simulink model "IFM_ModelComposer"  (R2024b)
settings: Solver=VariableStepAuto  StartTime=0.0  StopTime=2e-4  RelTol=1e-3
PreLoadFcn:
  | addpath('../Matlab_Scripts/','-end')
  | addpath('../System_Inputs/','-end')
  | System
undefined symbols (not defined in the file): Fs, time_delays, xlfda_numerator
libraries: hdlBasic x77, hdlDSPIP x4, hdlUtilities x1, vmcUtilities x1
settings Model: Creator=fsy  LastModifiedBy=fsydere

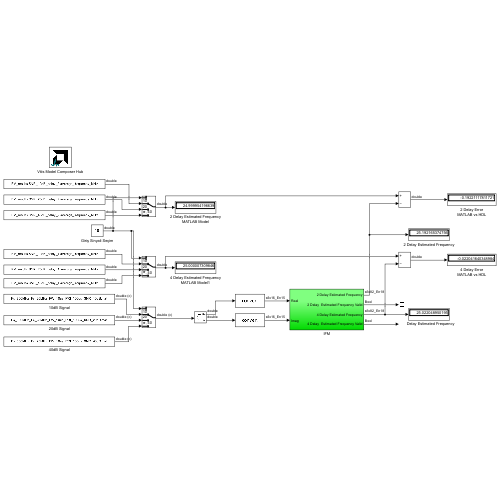
[thumbnail: Simulink's stored preview of the top-level diagram]
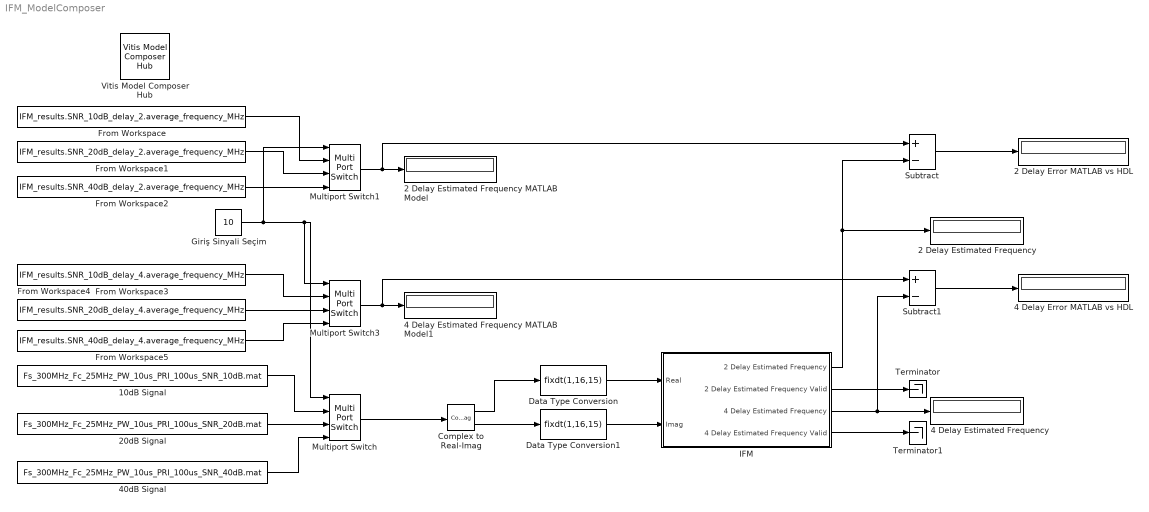
== system IFM_ModelComposer ==
  10dB Signal : FromFile  FileName=Fs_300MHz_Fc_25MHz_PW_10us_PRI_100us_SNR_10dB.mat  SampleTime=1/Fs
  2 Delay Error MATLAB vs HDL : Display
  2 Delay Estimated Frequency : Display
  2 Delay Estimated Frequency MATLAB Model : Display
  20dB Signal : FromFile  FileName=Fs_300MHz_Fc_25MHz_PW_10us_PRI_100us_SNR_20dB.mat  SampleTime=1/Fs
  4 Delay Error MATLAB vs HDL : Display
  4 Delay Estimated Frequency : Display
  4 Delay Estimated Frequency MATLAB Model1 : Display
  40dB Signal : FromFile  FileName=Fs_300MHz_Fc_25MHz_PW_10us_PRI_100us_SNR_40dB.mat  SampleTime=1/Fs
  Complex to Real-Imag : ComplexToRealImag
  Data Type Conversion : DataTypeConversion  OutDataTypeStr=fixdt(1,16,15)  RndMeth=Round
  Data Type Conversion1 : DataTypeConversion  OutDataTypeStr=fixdt(1,16,15)  RndMeth=Round
  From Workspace : FromWorkspace  VariableName=IFM_results.SNR_10dB_delay_2.average_frequency_MHz  SampleTime=1/Fs
  From Workspace1 : FromWorkspace  VariableName=IFM_results.SNR_20dB_delay_2.average_frequency_MHz  SampleTime=1/Fs
  From Workspace2 : FromWorkspace  VariableName=IFM_results.SNR_40dB_delay_2.average_frequency_MHz  SampleTime=1/Fs
  From Workspace3 : FromWorkspace  VariableName=IFM_results.SNR_10dB_delay_4.average_frequency_MHz  SampleTime=1/Fs
  From Workspace4 : FromWorkspace  VariableName=IFM_results.SNR_20dB_delay_4.average_frequency_MHz  SampleTime=1/Fs
  From Workspace5 : FromWorkspace  VariableName=IFM_results.SNR_40dB_delay_4.average_frequency_MHz  SampleTime=1/Fs
  Giriş Sinyali Seçim : Constant  Value=10  SampleTime=1/Fs
  IFM : Subsystem
  Multiport Switch : MultiPortSwitch  DataPortOrder=Specify indices  DataPortIndices={10,20,40}  OutDataTypeStr=double  SaturateOnIntegerOverflow=off  InputSameDT=off
  Multiport Switch1 : MultiPortSwitch  DataPortOrder=Specify indices  DataPortIndices={10,20,40}  OutDataTypeStr=double  SaturateOnIntegerOverflow=off  InputSameDT=off
  Multiport Switch3 : MultiPortSwitch  DataPortOrder=Specify indices  DataPortIndices={10,20,40}  OutDataTypeStr=double  SaturateOnIntegerOverflow=off  InputSameDT=off
  Subtract : Sum  Inputs=+-
  Subtract1 : Sum  Inputs=+-
  Terminator : Terminator
  Terminator1 : Terminator
  Vitis Model Composer Hub : vmcUtilities/Vitis Model Composer Hub  Tag=genX  CodeGeneration=off  SubsystemName=IFM  BlockHierPath=IFM_ModelComposer/IFM  CompilationType=HDLCompilation  SubsystemType=HDLNode  ExportTypeV2=IP Catalog  StartColumn=1  NumberOfColumns=1  TargetDirectory=./netlist  exportDesign=off  analyzeDesign=on  validateDesignOnHw=off  ExportType=AI Engines  IpVendor=xilinx.com  IpLibrary=hls  IpVersion=1.0  IpHWLanguage=Verilog  AieCompilerOptions={}  AieSimulatorOptions={}  CreateTestbench=on  TestbenchStackSize=10  RunRtlSim=off  RunCSim=off  RunAieSim=off  AieSimTimeout=50000  RunAieSimProfiling=off  LaunchVitisAnalyzer=off  PlotOutput=off  RunX86Sim=off  X86SimTimeout=10  GenHwImage=off  GenLibadfXo=off  GenHwValidationCode=off  PlatformType=Not Specified  HwSystemType=Baremetal  HwValidationTarget=hw  ProjDevice=Zynq UltraScale+ ZCU102 Evaluation Board (xczu9eg-ffvb1156-2-e)  ProjDevicePart=xczu9eg-ffvb1156-2-e  AIEType=None  SamplePeriod=-1  ClockFrequency=200  DataPathParallelism=1  xilinxfamily=zynquplus  part=xczu9eg  speed=-2-e  package=ffvb1156  directory=./netlist\ip\IFM\src  testbench=on  incr_netlist=off  synthesis_tool=Vivado  clock_wrapper=Clock Enables  dbl_ovrd=According to Block Masks  dcm_input_clock_period=10  sysclk_period=1e9/Fs  simulink_period=1/Fs  eval_field=0  IPInfoJsonString="{\"DUTSubsystemName\":\"IFM\",\"HDLSubsystem\":{\"SubsystemName\":\"IFM\",\"IPName\":\"IFM\",\"IPLibrary\":\"VMC\",\"IPVendor\":\"FSY\",\"IPVersion\":\"1.0\",\"TargetDirectory\":\"./netlist\",\"SubsystemDir\":\"./netlist\\\\ip\\\\IFM\",\"FreqHz\":\"300000000\"},\"SubsystemTag\":\"HDLNode\"}"  LogFileName=C:\Users\fsydere\Workspace\IFM\Model_Composer\netlist\model_composer.log  NThreads=10  IPConfigFile=C:\Users\fsydere\AppData\Local\Temp\vmctmp-16672868257368253290\IFM_ModelComposer_ipconfig.json
  wires:
  From Workspace/1 -> Multiport Switch1/2
  10dB Signal/1 -> Multiport Switch/2
  From Workspace5/1 -> Multiport Switch3/4
  From Workspace1/1 -> Multiport Switch1/3
  From Workspace2/1 -> Multiport Switch1/4
  Giriş Sinyali Seçim/1 -> Multiport Switch/1, Multiport Switch3/1, Multiport Switch1/1
  From Workspace3/1 -> Multiport Switch3/2
  From Workspace4/1 -> Multiport Switch3/3
  20dB Signal/1 -> Multiport Switch/3
  40dB Signal/1 -> Multiport Switch/4
  Multiport Switch1/1 -> Subtract/1, 2 Delay Estimated Frequency MATLAB Model/1
  Multiport Switch3/1 -> Subtract1/1, 4 Delay Estimated Frequency MATLAB Model1/1
  Multiport Switch/1 -> Complex to Real-Imag/1
  Complex to Real-Imag/1 -> Data Type Conversion/1
  Complex to Real-Imag/2 -> Data Type Conversion1/1
  Data Type Conversion/1 -> IFM/1(Real)
  Data Type Conversion1/1 -> IFM/2(Imag)
  Subtract1/1 -> 4 Delay Error MATLAB vs HDL/1
  IFM/1(2 Delay Estimated Frequency) -> 2 Delay Estimated Frequency/1, Subtract/2
  IFM/2(2 Delay Estimated Frequency Valid) -> Terminator/1
  IFM/3(4 Delay Estimated Frequency) -> Subtract1/2, 4 Delay Estimated Frequency/1
  IFM/4(4 Delay Estimated Frequency Valid) -> Terminator1/1
  Subtract/1 -> 2 Delay Error MATLAB vs HDL/1

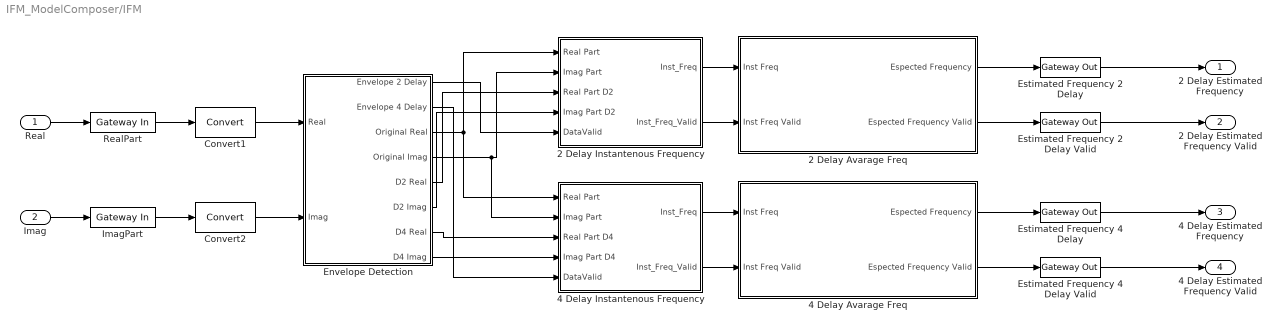
== system IFM_ModelComposer/IFM ==
  Real : Inport
  Imag : Inport  Port=2
  2 Delay Avarage Freq : Subsystem
  2 Delay Instantenous Frequency : Subsystem
  4 Delay Avarage Freq : Subsystem
  4 Delay Instantenous Frequency : Subsystem
  Convert1 : hdlBasic/Convert  gui_display_data_type=Fixed-point  arith_type=Signed (2's comp)  n_bits=16  bin_pt=15  float_type=Single  exp_bits=8  fraction_bits=24  quantization=Truncate  overflow=Wrap  en=off  latency=0  pipeline=off  XmcBlockStatus=1  maskContainerNames=group2  block_type=convert  block_config=sysgen:Convert_config  block_width=595  block_height=885
  Convert2 : hdlBasic/Convert  gui_display_data_type=Fixed-point  arith_type=Signed (2's comp)  n_bits=16  bin_pt=15  float_type=Single  exp_bits=8  fraction_bits=24  quantization=Truncate  overflow=Wrap  en=off  latency=0  pipeline=off  XmcBlockStatus=1  maskContainerNames=group2  block_type=convert  block_config=sysgen:Convert_config  block_width=595  block_height=885
  Envelope Detection : Subsystem
  Estimated Frequency 2 Delay : hdlBasic/Gateway Out  inherit_from_input=on  bool_to_boolean=off  hdl_port=on  rows=1  columns=1  UseAsDAC=off  DACChannel='1'  interface=None  automatic_assignment=on  address_offset=hex2dec('00')  intf_name=''  intf_description=''  timing_constraint=None  locs_specified=off  LOCs={}  io_standard={}  XmcBlockStatus=1  maskContainerNames=group4  block_type=gatewayout  block_config=sysgen:gateway_out_config  block_width_w=590  block_height_w=620  block_width=620  block_height=750
  Estimated Frequency 2 Delay Valid : hdlBasic/Gateway Out  inherit_from_input=on  bool_to_boolean=off  hdl_port=on  rows=1  columns=1  UseAsDAC=off  DACChannel='1'  interface=None  automatic_assignment=on  address_offset=hex2dec('00')  intf_name=''  intf_description=''  timing_constraint=None  locs_specified=off  LOCs={}  io_standard={}  XmcBlockStatus=1  maskContainerNames=group4  block_type=gatewayout  block_config=sysgen:gateway_out_config  block_width_w=590  block_height_w=620  block_width=620  block_height=750
  Estimated Frequency 4 Delay : hdlBasic/Gateway Out  inherit_from_input=on  bool_to_boolean=off  hdl_port=on  rows=1  columns=1  UseAsDAC=off  DACChannel='1'  interface=None  automatic_assignment=on  address_offset=hex2dec('00')  intf_name=''  intf_description=''  timing_constraint=None  locs_specified=off  LOCs={}  io_standard={}  XmcBlockStatus=1  maskContainerNames=group4  block_type=gatewayout  block_config=sysgen:gateway_out_config  block_width_w=590  block_height_w=620  block_width=620  block_height=750
  Estimated Frequency 4 Delay Valid : hdlBasic/Gateway Out  inherit_from_input=on  bool_to_boolean=off  hdl_port=on  rows=1  columns=1  UseAsDAC=off  DACChannel='1'  interface=None  automatic_assignment=on  address_offset=hex2dec('00')  intf_name=''  intf_description=''  timing_constraint=None  locs_specified=off  LOCs={}  io_standard={}  XmcBlockStatus=1  maskContainerNames=group4  block_type=gatewayout  block_config=sysgen:gateway_out_config  block_width_w=590  block_height_w=620  block_width=620  block_height=750
  ImagPart : hdlBasic/Gateway In  gui_display_data_type=Fixed-point  arith_type=Signed (2's comp)  n_bits=16  bin_pt=15  preci_type=Single  exp_width=8  frac_width=24  rows=1  columns=1  quantization=Truncate  overflow=Wrap  period=1/Fs  UseAsADC=off  ADCChannel='1'  interface=None  automatic_assignment=on  address_offset=hex2dec('00')  intf_name=''  intf_description=''  default_value=0  timing_constraint=None  locs_specified=off  LOCs={}  io_standard={}  inherit_from_input=off  hdl_port=on  XmcBlockStatus=1  maskContainerNames=group4  block_type=gatewayin  block_config=sysgen:gateway_in_config  block_width_w=590  block_height_w=620  block_width=640  block_height=850
  RealPart : hdlBasic/Gateway In  gui_display_data_type=Fixed-point  arith_type=Signed (2's comp)  n_bits=16  bin_pt=15  preci_type=Single  exp_width=8  frac_width=24  rows=1  columns=1  quantization=Truncate  overflow=Wrap  period=1/Fs  UseAsADC=off  ADCChannel='1'  interface=None  automatic_assignment=on  address_offset=hex2dec('00')  intf_name=''  intf_description=''  default_value=0  timing_constraint=None  locs_specified=off  LOCs={}  io_standard={}  inherit_from_input=off  hdl_port=on  XmcBlockStatus=1  maskContainerNames=group4  block_type=gatewayin  block_config=sysgen:gateway_in_config  block_width_w=590  block_height_w=620  block_width=640  block_height=850
  2 Delay Estimated Frequency : Outport
  2 Delay Estimated Frequency Valid : Outport  Port=2
  4 Delay Estimated Frequency : Outport  Port=3
  4 Delay Estimated Frequency Valid : Outport  Port=4
  wires:
  2 Delay Avarage Freq/1(Espected Frequency) -> Estimated Frequency 2 Delay/1
  Real/1 -> RealPart/1
  ImagPart/1 -> Convert2/1
  Imag/1 -> ImagPart/1
  RealPart/1 -> Convert1/1
  Convert2/1 -> Envelope Detection/2(Imag)
  Envelope Detection/3(Original Real) -> 4 Delay Instantenous Frequency/1(Real Part), 2 Delay Instantenous Frequency/1(Real Part)
  Convert1/1 -> Envelope Detection/1(Real)
  Envelope Detection/1(Envelope 2 Delay) -> 2 Delay Instantenous Frequency/5(DataValid)
  Envelope Detection/2(Envelope 4 Delay) -> 4 Delay Instantenous Frequency/5(DataValid)
  Envelope Detection/4(Original Imag) -> 4 Delay Instantenous Frequency/2(Imag Part), 2 Delay Instantenous Frequency/2(Imag Part)
  Envelope Detection/5(D2 Real) -> 2 Delay Instantenous Frequency/3(Real Part D2)
  Envelope Detection/6(D2 Imag) -> 2 Delay Instantenous Frequency/4(Imag Part D2)
  Envelope Detection/7(D4 Real) -> 4 Delay Instantenous Frequency/3(Real Part D4)
  Envelope Detection/8(D4 Imag) -> 4 Delay Instantenous Frequency/4(Imag Part D4)
  2 Delay Instantenous Frequency/1(Inst_Freq) -> 2 Delay Avarage Freq/1(Inst Freq)
  2 Delay Instantenous Frequency/2(Inst_Freq_Valid) -> 2 Delay Avarage Freq/2(Inst Freq Valid)
  4 Delay Avarage Freq/2(Espected Frequency Valid) -> Estimated Frequency 4 Delay Valid/1
  4 Delay Instantenous Frequency/1(Inst_Freq) -> 4 Delay Avarage Freq/1(Inst Freq)
  4 Delay Instantenous Frequency/2(Inst_Freq_Valid) -> 4 Delay Avarage Freq/2(Inst Freq Valid)
  Estimated Frequency 2 Delay/1 -> 2 Delay Estimated Frequency/1
  2 Delay Avarage Freq/2(Espected Frequency Valid) -> Estimated Frequency 2 Delay Valid/1
  4 Delay Avarage Freq/1(Espected Frequency) -> Estimated Frequency 4 Delay/1
  Estimated Frequency 2 Delay Valid/1 -> 2 Delay Estimated Frequency Valid/1
  Estimated Frequency 4 Delay/1 -> 4 Delay Estimated Frequency/1
  Estimated Frequency 4 Delay Valid/1 -> 4 Delay Estimated Frequency Valid/1

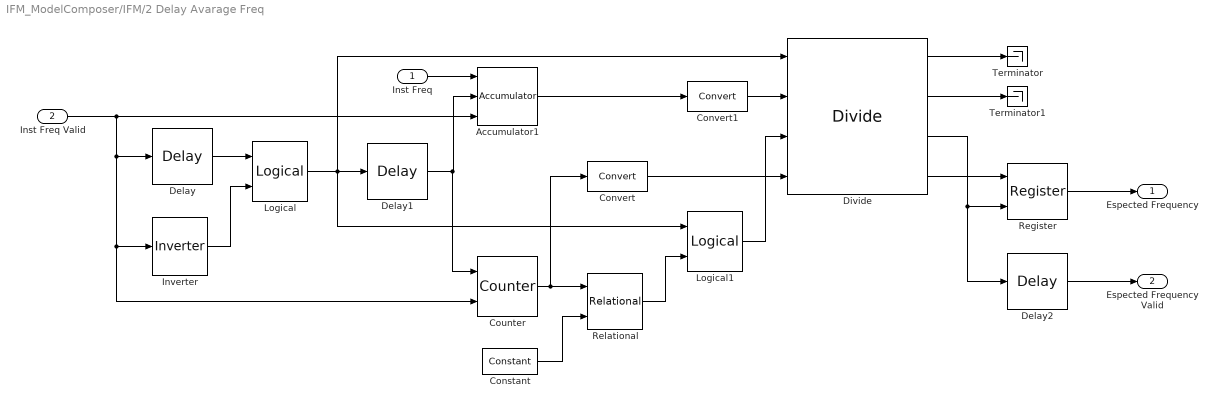
== system IFM_ModelComposer/IFM/2 Delay Avarage Freq ==
  Inst Freq : Inport
  Inst Freq Valid : Inport  Port=2
  Accumulator1 : hdlBasic/Accumulator  operation=Add  n_bits=64  overflow=Wrap  scale=1  rst=on  hasbypass=off  en=on  latency=1  msb_inp=100  msb=100  lsb=-100  use_behavioral_HDL=on  implementation=Fabric  XmcBlockStatus=1  maskContainerNames=group3  block_type=accum  block_config=sysgen:Accum_config  block_width=566  block_height=845
  Constant : hdlBasic/Constant  const=2  gui_display_data_type=Fixed-point  arith_type=Unsigned  n_bits=16  bin_pt=0  preci_type=Single  exp_width=8  frac_width=24  explicit_period=off  period=1  XmcBlockStatus=1  maskContainerNames=tabcontainer1  block_type=constant  block_config=sysgen:Constant_config
  Convert : hdlBasic/Convert  gui_display_data_type=Fixed-point  arith_type=Signed (2's comp)  n_bits=64  bin_pt=26  float_type=Single  exp_bits=8  fraction_bits=24  quantization=Truncate  overflow=Wrap  en=off  latency=0  pipeline=off  XmcBlockStatus=1  maskContainerNames=group2  block_type=convert  block_config=sysgen:Convert_config  block_width=595  block_height=885
  Convert1 : hdlBasic/Convert  gui_display_data_type=Fixed-point  arith_type=Signed (2's comp)  n_bits=64  bin_pt=26  float_type=Single  exp_bits=8  fraction_bits=24  quantization=Truncate  overflow=Wrap  en=off  latency=0  pipeline=off  XmcBlockStatus=1  maskContainerNames=group2  block_type=convert  block_config=sysgen:Convert_config  block_width=595  block_height=885
  Counter : hdlBasic/Counter  cnt_type=Free running  cnt_to=Inf  operation=Up  start_count=0  cnt_by_val=1  arith_type=Unsigned  n_bits=16  bin_pt=0  load_pin=off  rst=on  en=on  explicit_period=Explicit  period=1/Fs  use_behavioral_HDL=off  implementation=Fabric  XmcBlockStatus=1  maskContainerNames=group1  block_type=counter  block_config=sysgen:Counter_config  block_width=531  block_height=1023
  Delay : hdlBasic/Delay  rst=off  en=off  latency=1  reg_retiming=off  XmcBlockStatus=1  maskContainerNames=group1  block_type=delay  block_config=sysgen:Delay_config
  Delay1 : hdlBasic/Delay  rst=off  en=off  latency=1  reg_retiming=off  XmcBlockStatus=1  maskContainerNames=group1  block_type=delay  block_config=sysgen:Delay_config
  Delay2 : hdlBasic/Delay  rst=off  en=off  latency=1  reg_retiming=off  XmcBlockStatus=1  maskContainerNames=group1  block_type=delay  block_config=sysgen:Delay_config
  Divide : hdlBasic/Divide  flow_control=Blocking  axi_optimize_goal=Resources  algorithm_type=High_Radix  fractional_width=26  latency=1  rate=1  has_a_tlast=off  has_a_tuser=off  has_b_tlast=off  has_b_tuser=off  en=off  has_result_tready=off  result_tlast_behv=Pass_A_TLAST  has_underflow=off  has_overflow=off  has_invalid_op=off  has_divide_by_zero=off  fpo_op_type=mergeddivide  XmcBlockStatus=1  maskContainerNames=tabcontainer1  block_type=divide  block_config=sysgen:FPOBlockDescriptor_config
  Inverter : hdlBasic/Inverter  en=off  latency=0  XmcBlockStatus=1  maskContainerNames=group2  block_type=inv  block_config=sysgen:Inverter_config
  Logical : hdlBasic/Logical  logical_function=AND  inputs=2  en=off  latency=0  precision=Full  arith_type=Unsigned  n_bits=16  bin_pt=0  align_bp=on  overflow=[]  quantization=[]  XmcBlockStatus=1  maskContainerNames=tabcontainer1  block_type=logical  block_config=sysgen:Logical_config
  Logical1 : hdlBasic/Logical  logical_function=AND  inputs=2  en=off  latency=0  precision=Full  arith_type=Unsigned  n_bits=16  bin_pt=0  align_bp=on  overflow=[]  quantization=[]  XmcBlockStatus=1  maskContainerNames=tabcontainer1  block_type=logical  block_config=sysgen:Logical_config
  Register : hdlBasic/Register  init=0  rst=off  en=on  XmcBlockStatus=1  maskContainerNames=tabcontainer1  block_type=register  block_config=sysgen:Register_config
  Relational : hdlBasic/Relational  mode=a>b  op_type=Bool  en=off  latency=0  XmcBlockStatus=1  maskContainerNames=tabcontainer1  block_type=relational  block_config=sysgen:Relational_config
  Terminator : Terminator
  Terminator1 : Terminator
  Espected Frequency : Outport
  Espected Frequency Valid : Outport  Port=2
  wires:
  Inst Freq/1 -> Accumulator1/1
  Inst Freq Valid/1 -> Counter/2, Inverter/1, Delay/1, Accumulator1/3
  Divide/3 -> Delay2/1, Register/2
  Delay1/1 -> Counter/1, Accumulator1/2
  Divide/4 -> Register/1
  Delay/1 -> Logical/1
  Register/1 -> Espected Frequency/1
  Logical1/1 -> Divide/3
  Inverter/1 -> Logical/2
  Logical/1 -> Divide/1, Delay1/1, Logical1/1
  Convert1/1 -> Divide/2
  Accumulator1/1 -> Convert1/1
  Counter/1 -> Relational/1, Convert/1
  Constant/1 -> Relational/2
  Relational/1 -> Logical1/2
  Convert/1 -> Divide/4
  Divide/1 -> Terminator/1
  Divide/2 -> Terminator1/1
  Delay2/1 -> Espected Frequency Valid/1

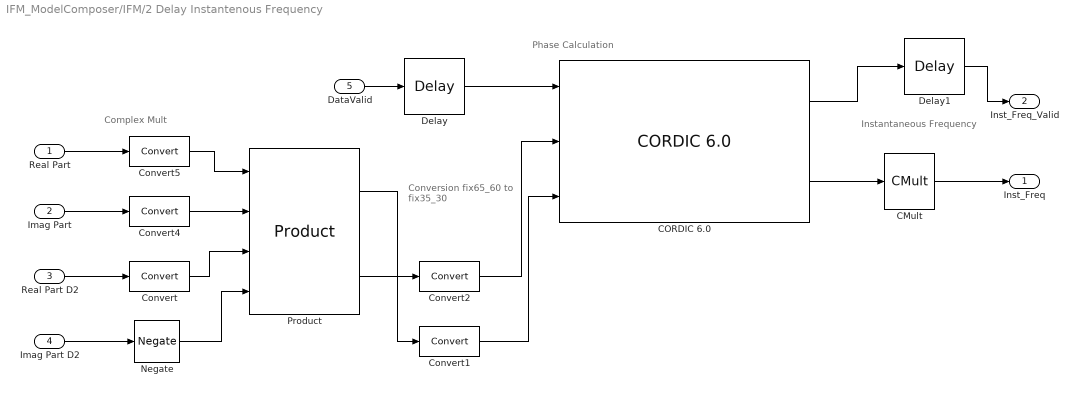
== system IFM_ModelComposer/IFM/2 Delay Instantenous Frequency ==
  note: Conversion
      | fix65_60
      | to
      | fix35_30
  note: Complex Mult
  note: Instantaneous
      | Frequency
  note: Phase Calculation
  Real Part : Inport
  Imag Part : Inport  Port=2
  Real Part D2 : Inport  Port=3
  Imag Part D2 : Inport  Port=4
  DataValid : Inport  Port=5
  CMult : hdlBasic/CMult  const=Fs/(2*pi*time_delays(1)*1e6)  gui_display_data_type=Fixed-point  const_n_bits=20  const_bin_pt=13  float_type=Single  exp_bits=8  fraction_bits=24  en=off  latency=1  precision=Full  arith_type="Signed  (2's comp)"  n_bits=16  bin_pt=14  quantization=Truncate  overflow=Wrap  use_behavioral_HDL=off  mem_type=Distributed RAM  pipeline=off  XmcBlockStatus=1  maskContainerNames=tabcontainer1  block_type=cmult  block_config=sysgen:CMult_config
      settings: infoedit=[]
  CORDIC 6.0 : hdlDSPIP/CORDIC 6.0   functional_selection=Arc_Tan  architectural_configuration=Parallel  pipelining_mode=Maximum  data_format=SignedFraction  phase_format=Radians  input_width=32  output_width=16  round_mode=Truncate  iterations=0  precision=0  compensation_scaling=No_Scale_Compensation  coarse_rotation=on  aclken=off  aresetn=off  out_tready=off  cartesian_has_tuser=off  cartesian_has_tlast=off  cartesian_tuser_width=1  phase_has_tuser=off  phase_has_tlast=off  phase_tuser_width=1  out_tlast_behv=Null  flow_control=NonBlocking  optimize_goal=Resources  trim_axipin_name=on  simulation_type=hybrid_sim  simulation_model=sysgen:cordic_v6_0  data_path_portlist={'s_axis_cartesian_tdata_imag', 's_axis_cartesian_tdata_real', 's_axis_phase_tdata_phase', 'm_axis_dout_tdata_imag', 'm_axis_dout_tdata_real', 'm_axis_dout_tdata_phase','m_axis_dout_tdata'}  ip_name=CORDIC  ip_version=6.0  dsptool_ready=true  ipcore_usecache=true  ipcore_useipmodelcache=true  wrapper_available=true  port_translation_map={ 'aclken' => 'en', 'aresetn' => 'rst' }  XmcBlockStatus=1  maskContainerNames=group15  block_type=cordic_v6_0  block_config=sysgen:rodinimport_config  block_width=800
  Convert : hdlBasic/Convert  gui_display_data_type=Fixed-point  arith_type="Signed  (2's comp)"  n_bits=32  bin_pt=30  float_type=Single  exp_bits=8  fraction_bits=24  quantization=Truncate  overflow=Wrap  en=off  latency=1  pipeline=off  XmcBlockStatus=1  maskContainerNames=group2  block_type=convert  block_config=sysgen:Convert_config  block_width=595  block_height=885
  Convert1 : hdlBasic/Convert  gui_display_data_type=Fixed-point  arith_type="Signed  (2's comp)"  n_bits=32  bin_pt=30  float_type=Single  exp_bits=8  fraction_bits=24  quantization=Truncate  overflow=Wrap  en=off  latency=0  pipeline=off  XmcBlockStatus=1  maskContainerNames=group2  block_type=convert  block_config=sysgen:Convert_config  block_width=595  block_height=885
  Convert2 : hdlBasic/Convert  gui_display_data_type=Fixed-point  arith_type="Signed  (2's comp)"  n_bits=32  bin_pt=30  float_type=Single  exp_bits=8  fraction_bits=24  quantization=Truncate  overflow=Wrap  en=off  latency=0  pipeline=off  XmcBlockStatus=1  maskContainerNames=group2  block_type=convert  block_config=sysgen:Convert_config  block_width=595  block_height=885
  Convert4 : hdlBasic/Convert  gui_display_data_type=Fixed-point  arith_type="Signed  (2's comp)"  n_bits=32  bin_pt=30  float_type=Single  exp_bits=8  fraction_bits=24  quantization=Truncate  overflow=Wrap  en=off  latency=1  pipeline=off  XmcBlockStatus=1  maskContainerNames=group2  block_type=convert  block_config=sysgen:Convert_config  block_width=595  block_height=885
  Convert5 : hdlBasic/Convert  gui_display_data_type=Fixed-point  arith_type="Signed  (2's comp)"  n_bits=32  bin_pt=30  float_type=Single  exp_bits=8  fraction_bits=24  quantization=Truncate  overflow=Wrap  en=off  latency=1  pipeline=off  XmcBlockStatus=1  maskContainerNames=group2  block_type=convert  block_config=sysgen:Convert_config  block_width=595  block_height=885
  Delay : hdlBasic/Delay  rst=off  en=off  latency=5  reg_retiming=off  XmcBlockStatus=1  maskContainerNames=group1  block_type=delay  block_config=sysgen:Delay_config
  Delay1 : hdlBasic/Delay  rst=off  en=off  latency=1  reg_retiming=off  XmcBlockStatus=1  maskContainerNames=group1  block_type=delay  block_config=sysgen:Delay_config
  Negate : hdlBasic/Negate  precision=User Defined  arith_type="Signed  (2's comp)"  n_bits=32  bin_pt=30  quantization=Truncate  overflow=Wrap  en=off  latency=1  XmcBlockStatus=1  maskContainerNames=tabcontainer1  block_type=negate  block_config=sysgen:Negate_config
  Product : hdlBasic/Product  complex_multiplier=on  optimizegoal=Performance  simulation_type=fast_sim  simulation_model=sysgen:product_macro  XmcBlockStatus=1  maskContainerNames=<empty>  block_type=product_macro  block_config=sysgen:ProductMacro_config
  Inst_Freq : Outport
  Inst_Freq_Valid : Outport  Port=2
  wires:
  Convert/1 -> Product/3
  Convert5/1 -> Product/1
  Negate/1 -> Product/4
  Convert4/1 -> Product/2
  DataValid/1 -> Delay/1
  Delay1/1 -> Inst_Freq_Valid/1
  Imag Part/1 -> Convert4/1
  Convert2/1 -> CORDIC 6.0/2
  Convert1/1 -> CORDIC 6.0/3
  CORDIC 6.0/1 -> Delay1/1
  CORDIC 6.0/2 -> CMult/1
  Product/1 -> Convert1/1
  Product/2 -> Convert2/1
  CMult/1 -> Inst_Freq/1
  Real Part/1 -> Convert5/1
  Real Part D2/1 -> Convert/1
  Imag Part D2/1 -> Negate/1
  Delay/1 -> CORDIC 6.0/1

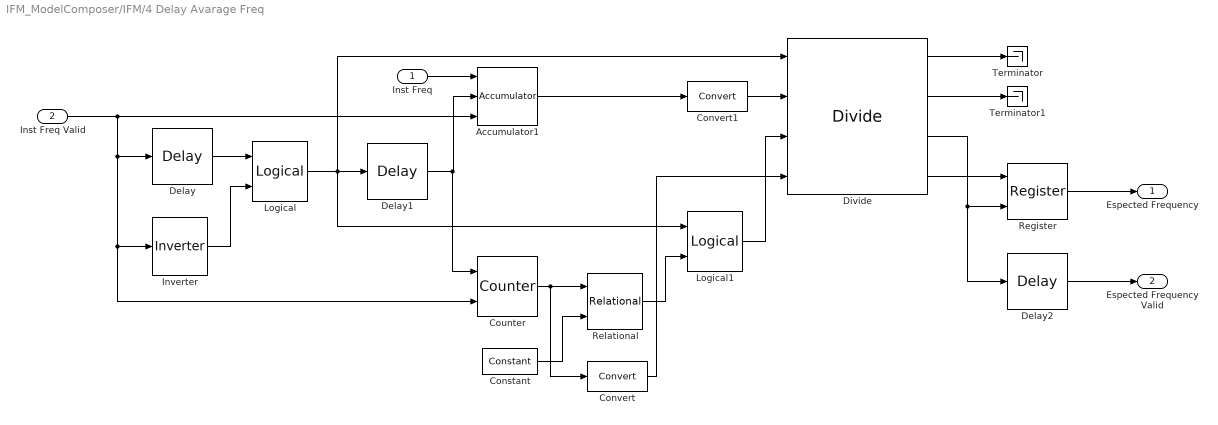
== system IFM_ModelComposer/IFM/4 Delay Avarage Freq ==
  Inst Freq : Inport
  Inst Freq Valid : Inport  Port=2
  Accumulator1 : hdlBasic/Accumulator  operation=Add  n_bits=64  overflow=Wrap  scale=1  rst=on  hasbypass=off  en=on  latency=1  msb_inp=100  msb=100  lsb=-100  use_behavioral_HDL=on  implementation=Fabric  XmcBlockStatus=1  maskContainerNames=group3  block_type=accum  block_config=sysgen:Accum_config  block_width=566  block_height=845
  Constant : hdlBasic/Constant  const=4  gui_display_data_type=Fixed-point  arith_type=Unsigned  n_bits=16  bin_pt=0  preci_type=Single  exp_width=8  frac_width=24  explicit_period=off  period=1  XmcBlockStatus=1  maskContainerNames=tabcontainer1  block_type=constant  block_config=sysgen:Constant_config
  Convert : hdlBasic/Convert  gui_display_data_type=Fixed-point  arith_type="Signed  (2's comp)"  n_bits=64  bin_pt=26  float_type=Single  exp_bits=8  fraction_bits=24  quantization=Truncate  overflow=Wrap  en=off  latency=0  pipeline=off  XmcBlockStatus=1  maskContainerNames=group2  block_type=convert  block_config=sysgen:Convert_config  block_width=595  block_height=885
  Convert1 : hdlBasic/Convert  gui_display_data_type=Fixed-point  arith_type="Signed  (2's comp)"  n_bits=64  bin_pt=26  float_type=Single  exp_bits=8  fraction_bits=24  quantization=Truncate  overflow=Wrap  en=off  latency=0  pipeline=off  XmcBlockStatus=1  maskContainerNames=group2  block_type=convert  block_config=sysgen:Convert_config  block_width=595  block_height=885
  Counter : hdlBasic/Counter  cnt_type=Free running  cnt_to=Inf  operation=Up  start_count=0  cnt_by_val=1  arith_type=Unsigned  n_bits=16  bin_pt=0  load_pin=off  rst=on  en=on  explicit_period=Explicit  period=1/Fs  use_behavioral_HDL=off  implementation=Fabric  XmcBlockStatus=1  maskContainerNames=group1  block_type=counter  block_config=sysgen:Counter_config  block_width=531  block_height=1023
  Delay : hdlBasic/Delay  rst=off  en=off  latency=1  reg_retiming=off  XmcBlockStatus=1  maskContainerNames=group1  block_type=delay  block_config=sysgen:Delay_config
  Delay1 : hdlBasic/Delay  rst=off  en=off  latency=1  reg_retiming=off  XmcBlockStatus=1  maskContainerNames=group1  block_type=delay  block_config=sysgen:Delay_config
  Delay2 : hdlBasic/Delay  rst=off  en=off  latency=1  reg_retiming=off  XmcBlockStatus=1  maskContainerNames=group1  block_type=delay  block_config=sysgen:Delay_config
  Divide : hdlBasic/Divide  flow_control=Blocking  axi_optimize_goal=Resources  algorithm_type=High_Radix  fractional_width=26  latency=1  rate=1  has_a_tlast=off  has_a_tuser=off  has_b_tlast=off  has_b_tuser=off  en=off  has_result_tready=off  result_tlast_behv=Pass_A_TLAST  has_underflow=off  has_overflow=off  has_invalid_op=off  has_divide_by_zero=off  fpo_op_type=mergeddivide  XmcBlockStatus=1  maskContainerNames=tabcontainer1  block_type=divide  block_config=sysgen:FPOBlockDescriptor_config
  Inverter : hdlBasic/Inverter  en=off  latency=0  XmcBlockStatus=1  maskContainerNames=group2  block_type=inv  block_config=sysgen:Inverter_config
  Logical : hdlBasic/Logical  logical_function=AND  inputs=2  en=off  latency=0  precision=Full  arith_type=Unsigned  n_bits=16  bin_pt=0  align_bp=on  overflow=[]  quantization=[]  XmcBlockStatus=1  maskContainerNames=tabcontainer1  block_type=logical  block_config=sysgen:Logical_config
  Logical1 : hdlBasic/Logical  logical_function=AND  inputs=2  en=off  latency=0  precision=Full  arith_type=Unsigned  n_bits=16  bin_pt=0  align_bp=on  overflow=[]  quantization=[]  XmcBlockStatus=1  maskContainerNames=tabcontainer1  block_type=logical  block_config=sysgen:Logical_config
  Register : hdlBasic/Register  init=0  rst=off  en=on  XmcBlockStatus=1  maskContainerNames=tabcontainer1  block_type=register  block_config=sysgen:Register_config
  Relational : hdlBasic/Relational  mode=a>b  op_type=Bool  en=off  latency=0  XmcBlockStatus=1  maskContainerNames=tabcontainer1  block_type=relational  block_config=sysgen:Relational_config
  Terminator : Terminator
  Terminator1 : Terminator
  Espected Frequency : Outport
  Espected Frequency Valid : Outport  Port=2
  wires:
  Inst Freq/1 -> Accumulator1/1
  Inst Freq Valid/1 -> Counter/2, Inverter/1, Delay/1, Accumulator1/3
  Divide/3 -> Delay2/1, Register/2
  Delay1/1 -> Counter/1, Accumulator1/2
  Divide/4 -> Register/1
  Delay/1 -> Logical/1
  Register/1 -> Espected Frequency/1
  Logical1/1 -> Divide/3
  Inverter/1 -> Logical/2
  Logical/1 -> Divide/1, Delay1/1, Logical1/1
  Convert1/1 -> Divide/2
  Accumulator1/1 -> Convert1/1
  Counter/1 -> Relational/1, Convert/1
  Constant/1 -> Relational/2
  Relational/1 -> Logical1/2
  Convert/1 -> Divide/4
  Divide/1 -> Terminator/1
  Divide/2 -> Terminator1/1
  Delay2/1 -> Espected Frequency Valid/1

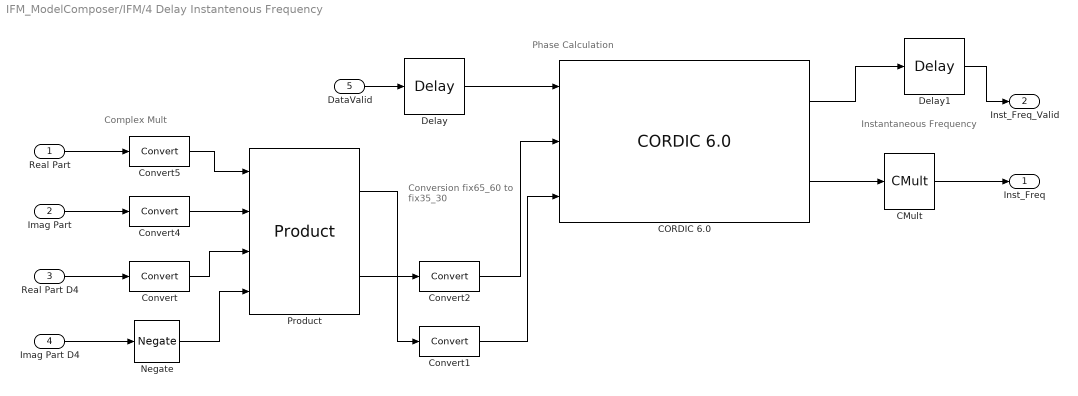
== system IFM_ModelComposer/IFM/4 Delay Instantenous Frequency ==
  note: Conversion
      | fix65_60
      | to
      | fix35_30
  note: Complex Mult
  note: Instantaneous
      | Frequency
  note: Phase Calculation
  Real Part : Inport
  Imag Part : Inport  Port=2
  Real Part D4 : Inport  Port=3
  Imag Part D4 : Inport  Port=4
  DataValid : Inport  Port=5
  CMult : hdlBasic/CMult  const=Fs/(2*pi*time_delays(2)*1e6)  gui_display_data_type=Fixed-point  const_n_bits=20  const_bin_pt=13  float_type=Single  exp_bits=8  fraction_bits=24  en=off  latency=1  precision=Full  arith_type="Signed  (2's comp)"  n_bits=16  bin_pt=14  quantization=Truncate  overflow=Wrap  use_behavioral_HDL=off  mem_type=Distributed RAM  pipeline=off  XmcBlockStatus=1  maskContainerNames=tabcontainer1  block_type=cmult  block_config=sysgen:CMult_config
      settings: infoedit=[]
  CORDIC 6.0 : hdlDSPIP/CORDIC 6.0   functional_selection=Arc_Tan  architectural_configuration=Parallel  pipelining_mode=Maximum  data_format=SignedFraction  phase_format=Radians  input_width=32  output_width=16  round_mode=Truncate  iterations=0  precision=0  compensation_scaling=No_Scale_Compensation  coarse_rotation=on  aclken=off  aresetn=off  out_tready=off  cartesian_has_tuser=off  cartesian_has_tlast=off  cartesian_tuser_width=1  phase_has_tuser=off  phase_has_tlast=off  phase_tuser_width=1  out_tlast_behv=Null  flow_control=NonBlocking  optimize_goal=Resources  trim_axipin_name=on  simulation_type=hybrid_sim  simulation_model=sysgen:cordic_v6_0  data_path_portlist={'s_axis_cartesian_tdata_imag', 's_axis_cartesian_tdata_real', 's_axis_phase_tdata_phase', 'm_axis_dout_tdata_imag', 'm_axis_dout_tdata_real', 'm_axis_dout_tdata_phase','m_axis_dout_tdata'}  ip_name=CORDIC  ip_version=6.0  dsptool_ready=true  ipcore_usecache=true  ipcore_useipmodelcache=true  wrapper_available=true  port_translation_map={ 'aclken' => 'en', 'aresetn' => 'rst' }  XmcBlockStatus=1  maskContainerNames=group15  block_type=cordic_v6_0  block_config=sysgen:rodinimport_config  block_width=800
  Convert : hdlBasic/Convert  gui_display_data_type=Fixed-point  arith_type="Signed  (2's comp)"  n_bits=32  bin_pt=30  float_type=Single  exp_bits=8  fraction_bits=24  quantization=Truncate  overflow=Wrap  en=off  latency=1  pipeline=off  XmcBlockStatus=1  maskContainerNames=group2  block_type=convert  block_config=sysgen:Convert_config  block_width=595  block_height=885
  Convert1 : hdlBasic/Convert  gui_display_data_type=Fixed-point  arith_type="Signed  (2's comp)"  n_bits=32  bin_pt=30  float_type=Single  exp_bits=8  fraction_bits=24  quantization=Truncate  overflow=Wrap  en=off  latency=0  pipeline=off  XmcBlockStatus=1  maskContainerNames=group2  block_type=convert  block_config=sysgen:Convert_config  block_width=595  block_height=885
  Convert2 : hdlBasic/Convert  gui_display_data_type=Fixed-point  arith_type="Signed  (2's comp)"  n_bits=32  bin_pt=30  float_type=Single  exp_bits=8  fraction_bits=24  quantization=Truncate  overflow=Wrap  en=off  latency=0  pipeline=off  XmcBlockStatus=1  maskContainerNames=group2  block_type=convert  block_config=sysgen:Convert_config  block_width=595  block_height=885
  Convert4 : hdlBasic/Convert  gui_display_data_type=Fixed-point  arith_type="Signed  (2's comp)"  n_bits=32  bin_pt=30  float_type=Single  exp_bits=8  fraction_bits=24  quantization=Truncate  overflow=Wrap  en=off  latency=1  pipeline=off  XmcBlockStatus=1  maskContainerNames=group2  block_type=convert  block_config=sysgen:Convert_config  block_width=595  block_height=885
  Convert5 : hdlBasic/Convert  gui_display_data_type=Fixed-point  arith_type="Signed  (2's comp)"  n_bits=32  bin_pt=30  float_type=Single  exp_bits=8  fraction_bits=24  quantization=Truncate  overflow=Wrap  en=off  latency=1  pipeline=off  XmcBlockStatus=1  maskContainerNames=group2  block_type=convert  block_config=sysgen:Convert_config  block_width=595  block_height=885
  Delay : hdlBasic/Delay  rst=off  en=off  latency=5  reg_retiming=off  XmcBlockStatus=1  maskContainerNames=group1  block_type=delay  block_config=sysgen:Delay_config
  Delay1 : hdlBasic/Delay  rst=off  en=off  latency=1  reg_retiming=off  XmcBlockStatus=1  maskContainerNames=group1  block_type=delay  block_config=sysgen:Delay_config
  Negate : hdlBasic/Negate  precision=User Defined  arith_type="Signed  (2's comp)"  n_bits=32  bin_pt=30  quantization=Truncate  overflow=Wrap  en=off  latency=1  XmcBlockStatus=1  maskContainerNames=tabcontainer1  block_type=negate  block_config=sysgen:Negate_config
  Product : hdlBasic/Product  complex_multiplier=on  optimizegoal=Performance  simulation_type=fast_sim  simulation_model=sysgen:product_macro  XmcBlockStatus=1  maskContainerNames=<empty>  block_type=product_macro  block_config=sysgen:ProductMacro_config
  Inst_Freq : Outport
  Inst_Freq_Valid : Outport  Port=2
  wires:
  Convert/1 -> Product/3
  Convert5/1 -> Product/1
  Negate/1 -> Product/4
  Convert4/1 -> Product/2
  DataValid/1 -> Delay/1
  Delay1/1 -> Inst_Freq_Valid/1
  Imag Part/1 -> Convert4/1
  Convert2/1 -> CORDIC 6.0/2
  Convert1/1 -> CORDIC 6.0/3
  CORDIC 6.0/1 -> Delay1/1
  CORDIC 6.0/2 -> CMult/1
  Product/1 -> Convert1/1
  Product/2 -> Convert2/1
  CMult/1 -> Inst_Freq/1
  Real Part/1 -> Convert5/1
  Real Part D4/1 -> Convert/1
  Imag Part D4/1 -> Negate/1
  Delay/1 -> CORDIC 6.0/1

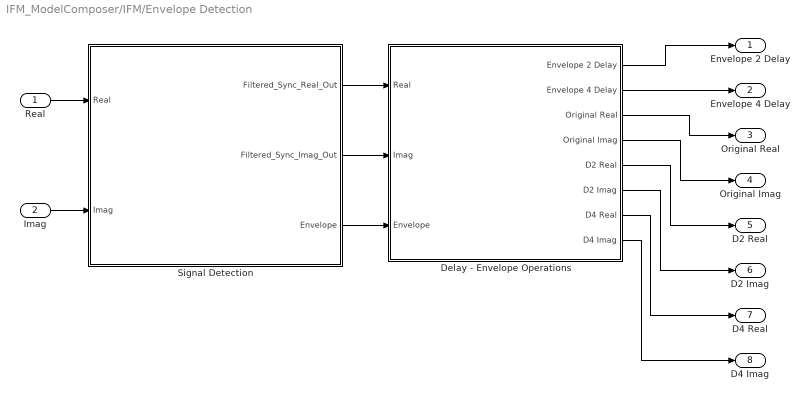
== system IFM_ModelComposer/IFM/Envelope Detection ==
  Real : Inport
  Imag : Inport  Port=2
  Delay - Envelope Operations : Subsystem
  Signal Detection : Subsystem
  Envelope 2 Delay : Outport
  Envelope 4 Delay : Outport  Port=2
  Original Real : Outport  Port=3
  Original Imag : Outport  Port=4
  D2 Real : Outport  Port=5
  D2 Imag : Outport  Port=6
  D4 Real : Outport  Port=7
  D4 Imag : Outport  Port=8
  wires:
  Imag/1 -> Signal Detection/2(Imag)
  Real/1 -> Signal Detection/1(Real)
  Signal Detection/1(Filtered_Sync_Real_Out) -> Delay - Envelope Operations/1(Real)
  Signal Detection/2(Filtered_Sync_Imag_Out) -> Delay - Envelope Operations/2(Imag)
  Delay - Envelope Operations/3(Original Real) -> Original Real/1
  Signal Detection/3(Envelope) -> Delay - Envelope Operations/3(Envelope)
  Delay - Envelope Operations/2(Envelope 4 Delay) -> Envelope 4 Delay/1
  Delay - Envelope Operations/1(Envelope 2 Delay) -> Envelope 2 Delay/1
  Delay - Envelope Operations/4(Original Imag) -> Original Imag/1
  Delay - Envelope Operations/5(D2 Real) -> D2 Real/1
  Delay - Envelope Operations/6(D2 Imag) -> D2 Imag/1
  Delay - Envelope Operations/7(D4 Real) -> D4 Real/1
  Delay - Envelope Operations/8(D4 Imag) -> D4 Imag/1

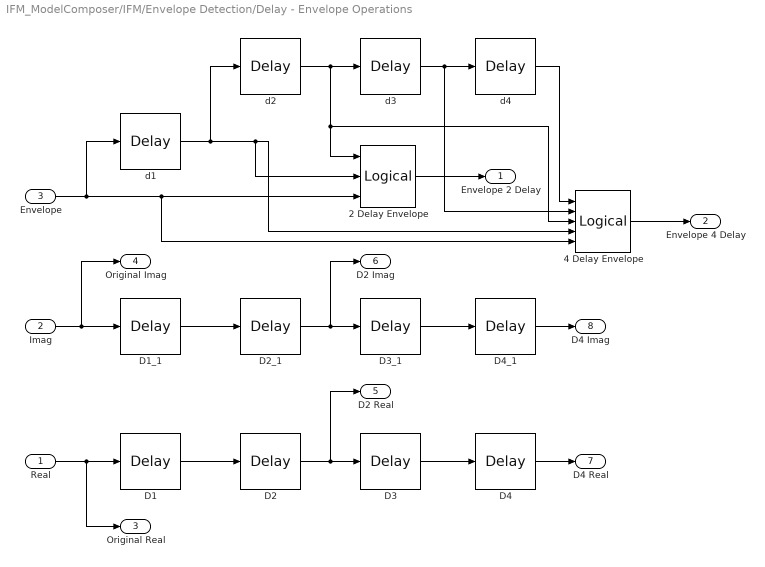
== system IFM_ModelComposer/IFM/Envelope Detection/Delay - Envelope Operations ==
  Real : Inport
  Imag : Inport  Port=2
  Envelope : Inport  Port=3
  2 Delay Envelope : hdlBasic/Logical  logical_function=AND  inputs=3  en=off  latency=0  precision=Full  arith_type=Unsigned  n_bits=16  bin_pt=0  align_bp=on  overflow=[]  quantization=[]  XmcBlockStatus=1  maskContainerNames=tabcontainer1  block_type=logical  block_config=sysgen:Logical_config
  4 Delay Envelope : hdlBasic/Logical  logical_function=AND  inputs=5  en=off  latency=0  precision=Full  arith_type=Unsigned  n_bits=16  bin_pt=0  align_bp=on  overflow=[]  quantization=[]  XmcBlockStatus=1  maskContainerNames=tabcontainer1  block_type=logical  block_config=sysgen:Logical_config
  D{1..4} (4 alike) : hdlBasic/Delay  rst=off  en=off  latency=1  reg_retiming=off  XmcBlockStatus=1  maskContainerNames=group1  block_type=delay  block_config=sysgen:Delay_config
  D1_1 : hdlBasic/Delay  rst=off  en=off  latency=1  reg_retiming=off  XmcBlockStatus=1  maskContainerNames=group1  block_type=delay  block_config=sysgen:Delay_config
  D2_1 : hdlBasic/Delay  rst=off  en=off  latency=1  reg_retiming=off  XmcBlockStatus=1  maskContainerNames=group1  block_type=delay  block_config=sysgen:Delay_config
  D3_1 : hdlBasic/Delay  rst=off  en=off  latency=1  reg_retiming=off  XmcBlockStatus=1  maskContainerNames=group1  block_type=delay  block_config=sysgen:Delay_config
  D4_1 : hdlBasic/Delay  rst=off  en=off  latency=1  reg_retiming=off  XmcBlockStatus=1  maskContainerNames=group1  block_type=delay  block_config=sysgen:Delay_config
  d{1..4} (4 alike) : hdlBasic/Delay  rst=off  en=off  latency=1  reg_retiming=off  XmcBlockStatus=1  maskContainerNames=group1  block_type=delay  block_config=sysgen:Delay_config
  Envelope 2 Delay : Outport
  Envelope 4 Delay : Outport  Port=2
  Original Real : Outport  Port=3
  Original Imag : Outport  Port=4
  D2 Real : Outport  Port=5
  D2 Imag : Outport  Port=6
  D4 Real : Outport  Port=7
  D4 Imag : Outport  Port=8
  wires:
  Envelope/1 -> 4 Delay Envelope/5, 2 Delay Envelope/3, d1/1
  D1/1 -> D2/1
  Real/1 -> D1/1, Original Real/1
  Imag/1 -> D1_1/1, Original Imag/1
  D2_1/1 -> D3_1/1, D2 Imag/1
  d2/1 -> 4 Delay Envelope/3, 2 Delay Envelope/1, d3/1
  D1_1/1 -> D2_1/1
  D4_1/1 -> D4 Imag/1
  d1/1 -> 2 Delay Envelope/2, 4 Delay Envelope/4, d2/1
  D2/1 -> D3/1, D2 Real/1
  d3/1 -> 4 Delay Envelope/2, d4/1
  2 Delay Envelope/1 -> Envelope 2 Delay/1
  D3_1/1 -> D4_1/1
  D3/1 -> D4/1
  d4/1 -> 4 Delay Envelope/1
  D4/1 -> D4 Real/1
  4 Delay Envelope/1 -> Envelope 4 Delay/1

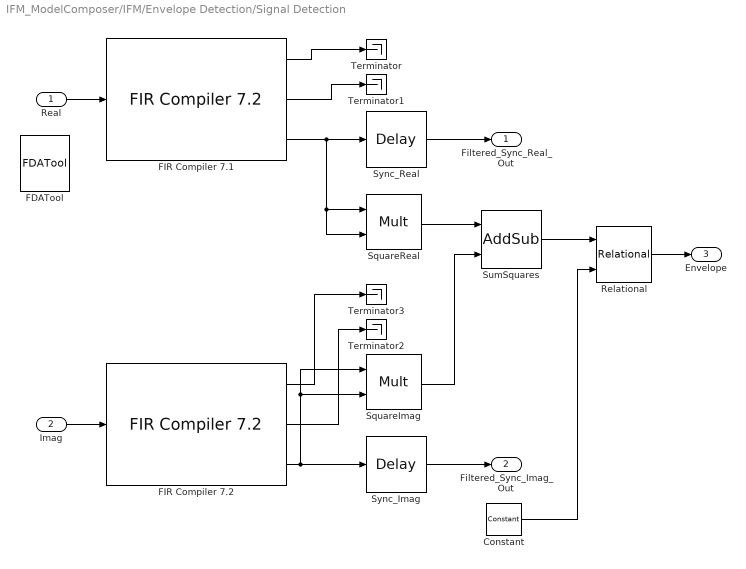
== system IFM_ModelComposer/IFM/Envelope Detection/Signal Detection ==
  Real : Inport
  Imag : Inport  Port=2
  Constant : hdlBasic/Constant  const=0.75  gui_display_data_type=Fixed-point  arith_type=Signed (2's comp)  n_bits=65  bin_pt=60  preci_type=Single  exp_width=8  frac_width=24  explicit_period=off  period=1  XmcBlockStatus=1  maskContainerNames=tabcontainer1  block_type=constant  block_config=sysgen:Constant_config
  FDATool : hdlUtilities/FDATool  block_type=fdatool
      settings: infoedit=FDATool
  FIR Compiler 7.1 : hdlDSPIP/FIR Compiler 7.2   coefficientvector=double(xlfda_numerator(strcat(bdroot,'/IFM/Envelope Detection/Signal Detection/FDATool')))  coefficient_sets=1  coefficient_reload=off  filter_type=Single_Rate  rate_change_type=Fixed_Fractional  interpolation_rate=1  decimation_rate=1  zero_pack_factor=1  channel_sequence=Basic  number_channels=1  pattern_list='P4-0,P4-1,P4-2,P4-3,P4-4'  number_paths=1  ratespecification=Maximum_Possible  sampleperiod=1  hardwareoversamplingrate=1  coefficient_sign=Unsigned  quantization=Quantize_Only  coefficient_width=16  bestprecision=off  coefficient_fractional_bits=15  coefficient_structure=Inferred  output_rounding_mode=Full_Precision  output_width=32  filter_architecture=Systolic_Multiply_Accumulate  optimization_goal=Area  optimization_list='None'  data_buffer_type=Automatic  coefficient_buffer_type=Automatic  input_buffer_type=Automatic  output_buffer_type=Automatic  preference_for_other_storage=Automatic  multi_column_support=Automatic  columnconfig='9'  inter_column_pipe_length=4  data_has_tlast=Not_Required  m_data_has_tready=off  s_data_has_fifo=off  s_data_has_tuser=Not_Required  m_data_has_tuser=Not_Required  s_config_sync_mode=On_Vector  s_config_method=Single  num_reload_slots=1  has_aclken=off  has_aresetn=off  reset_data_vector=on  trim_axipin_name=on  simulation_type=hybrid_sim  simulation_model=sysgen:xfirv7_2_cmodel  data_path_portlist={ 's_axis_data_tdata', 'm_axis_data_tdata' }  passband_min=0.0  passband_max=0.5  stopband_min=0.5  stopband_max=1.0  filter_selection=1  gui_behaviour='Sysgen_GUI'  data_sign=Signed  data_width=16  data_fractional_bits=0  data_tuser_width=1  wrapper_available=true  ip_wrap_arbitrary_binary_point=true  ip_name=FIR Compiler  ip_version=7.2  dsptool_ready=true  ipcore_usecache=true  ipcore_useipmodelcache=true  port_translation_map={ 'aclken' => 'en', 'aresetn' => 'rst' }  run_core_at_system_period=true  ipcore_xco_need_fpga_part=true  ipcore_fpga_part=[]  XmcBlockStatus=1  maskContainerNames=tabcontainer1  block_type=fir_compiler_v7_2  block_config=sysgen:rodinimport_config  block_width=820  block_height=600
  FIR Compiler 7.2 : hdlDSPIP/FIR Compiler 7.2   coefficientvector=double(xlfda_numerator(strcat(bdroot,'/IFM/Envelope Detection/Signal Detection/FDATool')))  coefficient_sets=1  coefficient_reload=off  filter_type=Single_Rate  rate_change_type=Fixed_Fractional  interpolation_rate=1  decimation_rate=1  zero_pack_factor=1  channel_sequence=Basic  number_channels=1  pattern_list='P4-0,P4-1,P4-2,P4-3,P4-4'  number_paths=1  ratespecification=Maximum_Possible  sampleperiod=1  hardwareoversamplingrate=1  coefficient_sign=Unsigned  quantization=Quantize_Only  coefficient_width=16  bestprecision=off  coefficient_fractional_bits=15  coefficient_structure=Inferred  output_rounding_mode=Full_Precision  output_width=32  filter_architecture=Systolic_Multiply_Accumulate  optimization_goal=Area  optimization_list='None'  data_buffer_type=Automatic  coefficient_buffer_type=Automatic  input_buffer_type=Automatic  output_buffer_type=Automatic  preference_for_other_storage=Automatic  multi_column_support=Automatic  columnconfig='9'  inter_column_pipe_length=4  data_has_tlast=Not_Required  m_data_has_tready=off  s_data_has_fifo=off  s_data_has_tuser=Not_Required  m_data_has_tuser=Not_Required  s_config_sync_mode=On_Vector  s_config_method=Single  num_reload_slots=1  has_aclken=off  has_aresetn=off  reset_data_vector=on  trim_axipin_name=on  simulation_type=hybrid_sim  simulation_model=sysgen:xfirv7_2_cmodel  data_path_portlist={ 's_axis_data_tdata', 'm_axis_data_tdata' }  passband_min=0.0  passband_max=0.5  stopband_min=0.5  stopband_max=1.0  filter_selection=1  gui_behaviour='Sysgen_GUI'  data_sign=Signed  data_width=16  data_fractional_bits=0  data_tuser_width=1  wrapper_available=true  ip_wrap_arbitrary_binary_point=true  ip_name=FIR Compiler  ip_version=7.2  dsptool_ready=true  ipcore_usecache=true  ipcore_useipmodelcache=true  port_translation_map={ 'aclken' => 'en', 'aresetn' => 'rst' }  run_core_at_system_period=true  ipcore_xco_need_fpga_part=true  ipcore_fpga_part=[]  XmcBlockStatus=1  maskContainerNames=tabcontainer1  block_type=fir_compiler_v7_2  block_config=sysgen:rodinimport_config  block_width=820  block_height=600
  Relational : hdlBasic/Relational  mode=a>=b  op_type=Bool  en=off  latency=1  XmcBlockStatus=1  maskContainerNames=tabcontainer1  block_type=relational  block_config=sysgen:Relational_config
  SquareImag : hdlBasic/Mult  precision=Full  arith_type="Signed  (2's comp)"  n_bits=32  bin_pt=30  quantization="Round  (unbiased: +/- Inf)"  overflow=Saturate  en=off  latency=1  opt_float=off  fp_mult_usage=No Usage  use_behavioral_HDL=on  opt=Speed  use_embedded=on  optimum_pipeline=off  pipeline=on  use_rpm=on  placement_style=Triangular  XmcBlockStatus=1  maskContainerNames=group1  block_type=mult  block_config=sysgen:Mult_config  block_width=598  block_height=876
  SquareReal : hdlBasic/Mult  precision=Full  arith_type="Signed  (2's comp)"  n_bits=32  bin_pt=30  quantization="Round  (unbiased: +/- Inf)"  overflow=Saturate  en=off  latency=1  opt_float=off  fp_mult_usage=No Usage  use_behavioral_HDL=on  opt=Speed  use_embedded=on  optimum_pipeline=off  pipeline=on  use_rpm=on  placement_style=Triangular  XmcBlockStatus=1  maskContainerNames=group1  block_type=mult  block_config=sysgen:Mult_config  block_width=598  block_height=876
  SumSquares : hdlBasic/AddSub  mode=Addition  use_carryin=off  use_carryout=off  en=off  latency=1  precision=Full  arith_type=Unsigned  n_bits=32  bin_pt=30  quantization=Truncate  overflow=Wrap  use_behavioral_HDL=on  hw_selection=Fabric  pipelined=off  XmcBlockStatus=1  maskContainerNames=tabcontainer1  block_type=addsub  block_config=sysgen:Addsub_config
  Sync_Imag : hdlBasic/Delay  rst=off  en=off  latency=3  reg_retiming=off  XmcBlockStatus=1  maskContainerNames=group1  block_type=delay  block_config=sysgen:Delay_config
  Sync_Real : hdlBasic/Delay  rst=off  en=off  latency=3  reg_retiming=off  XmcBlockStatus=1  maskContainerNames=group1  block_type=delay  block_config=sysgen:Delay_config
  Terminator{,1..3} (4 alike) : Terminator
  Filtered_Sync_Real_Out : Outport
  Filtered_Sync_Imag_Out : Outport  Port=2
  Envelope : Outport  Port=3
  wires:
  FIR Compiler 7.1/1 -> Terminator/1
  Imag/1 -> FIR Compiler 7.2/1
  Real/1 -> FIR Compiler 7.1/1
  SquareImag/1 -> SumSquares/2
  FIR Compiler 7.1/2 -> Terminator1/1
  Relational/1 -> Envelope/1
  FIR Compiler 7.1/3 -> SquareReal/2, SquareReal/1, Sync_Real/1
  FIR Compiler 7.2/3 -> SquareImag/1, SquareImag/2, Sync_Imag/1
  FIR Compiler 7.2/1 -> Terminator3/1
  FIR Compiler 7.2/2 -> Terminator2/1
  Sync_Real/1 -> Filtered_Sync_Real_Out/1
  SumSquares/1 -> Relational/1
  SquareReal/1 -> SumSquares/1
  Sync_Imag/1 -> Filtered_Sync_Imag_Out/1
  Constant/1 -> Relational/2
